simulink model "PRNDLController"  (R2025b)
settings: configuration reference "VehicleFixed1ms" (kept outside this file)
undefined symbols (not defined in the file): CtrlTcuDnShSpd, CtrlTcuUpShSpd, TireFrntWhlRadius, TireRearWhlRadius
libraries: autolibtranscontrolscommon x1
settings Model: DataDictionary=VirtualMotoTemplate.sldd  ModifiedByFormat=The MathWorks, Inc.  Creator=The MathWorks, Inc.  LastModifiedBy=The MathWorks, Inc.
settings ConfigSetRef: SourceName=VehicleFixed1ms

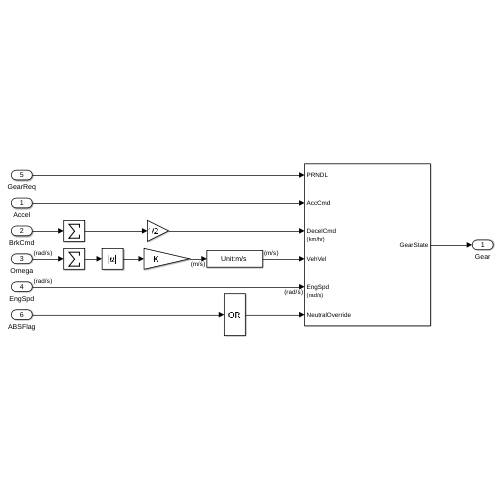
[thumbnail: Simulink's stored preview of the top-level diagram]
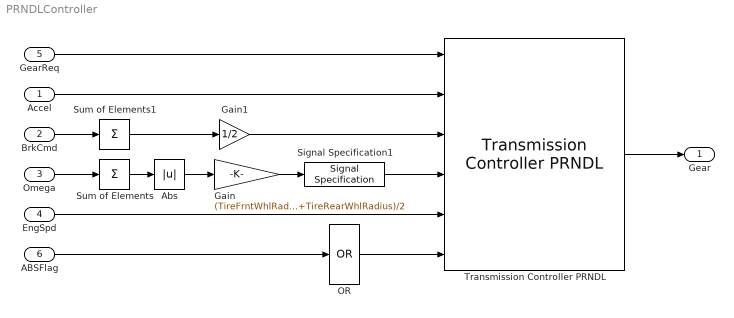
== system PRNDLController ==
  Accel : Inport  PortDimensions=1
  BrkCmd : Inport  Port=2  PortDimensions=2
  Omega : Inport  Port=3  Unit=rad/s  PortDimensions=2
  EngSpd : Inport  Port=4  Unit=rad/s
  GearReq : Inport  Port=5
  ABSFlag : Inport  Port=6  PortDimensions=2
  Abs : Abs  ZeroCross=off  SaturateOnIntegerOverflow=off
  Gain : Gain  Gain=(TireFrntWhlRadius+TireRearWhlRadius)/2
  Gain1 : Gain  Gain=1/2
  OR : Logic  Operator=OR  Inputs=1  AllPortsSameDT=off  OutDataTypeStr=boolean
  Signal Specification1 : SignalSpecification  Unit=m/s
  Sum of Elements : Sum  Inputs=+
  Sum of Elements1 : Sum  Inputs=+
  Transmission Controller PRNDL : autolibtranscontrolscommon/Transmission Controller PRNDL  DriveMode=off  GearInit=0  LugSpd=1200  MinUpSpd=2000  tClutchUp=.1  tClutchDn=.1  tPark=120  VelUnit=km/hr  UpShSpd=repmat(CtrlTcuUpShSpd,1,1,2)  UpLdBpt=CtrlTcuUpLdBpt  UpShBpt=1:7  UpPtBpt=[1 2]  DnShfSpd=repmat(CtrlTcuDnShSpd,1,1,2)  DnShSpd=[10 15 25 30 40 55 75; 10 18 25 35 50 65 80; 12 18 21 55 65 75 85; 15 20 25 55 70 80 95]  DnLdBpt=CtrlTcuDnLdBpt  DnShBpt=2:8  DnPtBpt=[1 2]  POFS=zeros(4,1)  GOFS=zeros(1,7)  Ngears=8  aMode=2
  Gear : Outport  VectorParamsAs1DForOutWhenUnconnected=off
  wires:
  Sum of Elements1/1 -> Gain1/1
  Gain/1 -> Signal Specification1/1
  Sum of Elements/1 -> Abs/1
  Accel/1 -> Transmission Controller PRNDL/2
  BrkCmd/1 -> Sum of Elements1/1
  Omega/1 -> Sum of Elements/1
  GearReq/1 -> Transmission Controller PRNDL/1
  Signal Specification1/1 -> Transmission Controller PRNDL/4
  Transmission Controller PRNDL/1 -> Gear/1
  Gain1/1 -> Transmission Controller PRNDL/3
  OR/1 -> Transmission Controller PRNDL/6
  EngSpd/1 -> Transmission Controller PRNDL/5
  ABSFlag/1 -> OR/1
  Abs/1 -> Gain/1
